simulink model "hydropower_plant"  (R2016a)
settings: Solver=VariableStepAuto  StartTime=0.0  StopTime=10.0  RelTol=1e-3
libraries: simulink x3
settings Model: Creator=desilvtk  LastModifiedBy=desilvtk

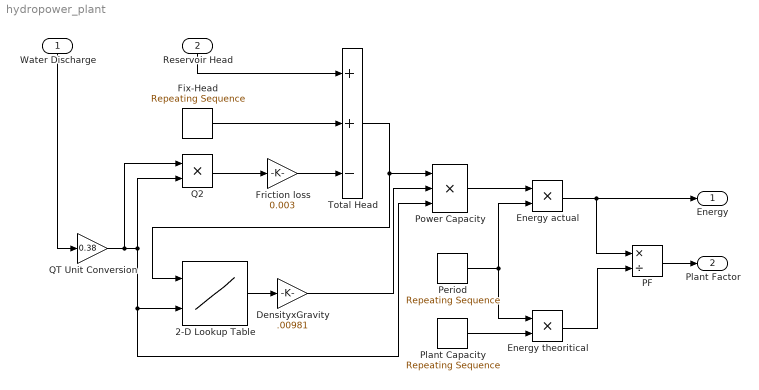
== system hydropower_plant ==
  Water Discharge : Inport
  Reservoir Head : Inport  Port=2
  2-D Lookup Table : Lookup_n-D  BreakpointsForDimension1=[130,150,170,190,210]  BreakpointsForDimension2=|  Table="[0.7790    0.8550    0.8550; 0.7980    0.9025    0.8740; 0.7980    0.9025    0.8835; 0.7885    0.9025    0.8740; 0.7885    0.8930    0.8740]"  InternalRulePriority=Speed  RndMeth=Simplest  InputSameDT=on
      | [41.6340,   83.2680,  124.9020
      | ]
  DensityxGravity : Gain  Gain=.00981
  Energy actual : Product
  Energy theoritical : Product
  Fix-Head : simulink/Sources/Repeating Sequence  rep_seq_t=[1,2,3,4,5,6,7,8,9,10,11,12]  rep_seq_y=[91,91,91,91,91,91,91,91,91,91,91,91]
  Friction loss : Gain  Gain=0.003
  PF : Product  Inputs=*/
  Period : simulink/Sources/Repeating Sequence  rep_seq_t=[1,2,3,4,5,6,7,8,9,10,11,12]  rep_seq_y=[0.72,.744,.720,.744,.744,.72,.744,.720,.744,.744,.672,.744]
  "Plant Capacity " : simulink/Sources/Repeating Sequence  rep_seq_t=[1,2,3,4,5,6,7,8,9,10,11,12]  rep_seq_y=[.18,.18,.18,.18,.18,.18,.18,.18,.18,.18,.18,.18]
  Power Capacity : Product  Inputs=3
  Q2 : Product
  QT Unit Conversion : Gain  Gain=0.38
  Total Head : Sum  Inputs=++-
  Energy : Outport
  Plant Factor : Outport  Port=2
  wires:
  Water Discharge/1 -> QT Unit Conversion/1
  Reservoir Head/1 -> Total Head/1
  QT Unit Conversion/1 -> Power Capacity/3, 2-D Lookup Table/2, Q2/2, Q2/1
  Q2/1 -> Friction loss/1
  Power Capacity/1 -> Energy actual/1
  Friction loss/1 -> Total Head/3
  Energy actual/1 -> Energy/1, PF/1
  Total Head/1 -> 2-D Lookup Table/1, Power Capacity/1
  Fix-Head/1 -> Total Head/2
  DensityxGravity/1 -> Power Capacity/2
  Period/1 -> Energy actual/2, Energy theoritical/1
  Energy theoritical/1 -> PF/2
  PF/1 -> Plant Factor/1
  2-D Lookup Table/1 -> DensityxGravity/1
  "Plant Capacity "/1 -> Energy theoritical/2
